simulink model "notch_filter"  (R2017a)
settings: Solver=VariableStepAuto  StartTime=0.0  StopTime=10  RelTol=1e-3
InitFcn:
  | r = 4700
  | c = 0.1e-6
  | fl = 1/(2*pi*r*c)
  | wl = 2*pi*fl
  | 
  | fn = 1526
  | wn = 2*pi*fn
  | 
  | t = 1.5e-4
libraries: dspstat3 x1, dspfdesign x1
settings Model: Creator=frede  LastModifiedBy=frede

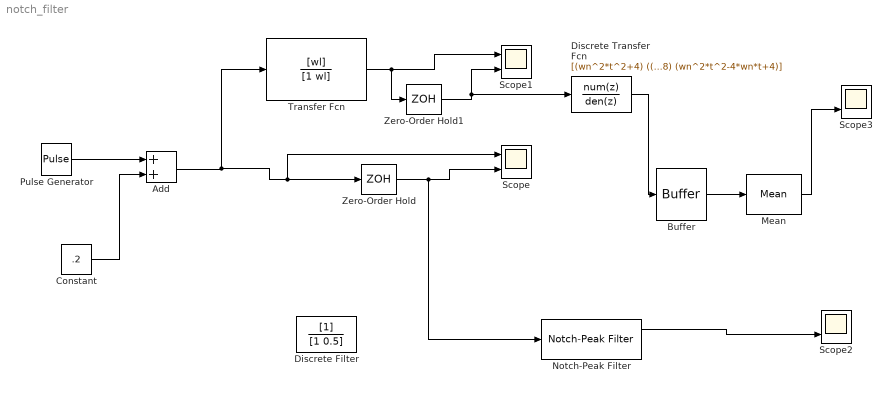
== system notch_filter ==
  Add : Sum
  Buffer : Buffer  N=230  OutputFrames=off
  Constant : Constant  Value=.2
  Discrete Transfer Fcn : DiscreteTransferFcn  Numerator=[(wn^2*t^2+4) ((wn^2*t-4)*2) (wn^2+4)]  Denominator=[(wn^2*t^2+4*wn*t+4) (2*wn^2*t^2-8) (wn^2*t^2-4*wn*t+4)]  SampleTime=t
  Discrete Filter : DiscreteFilter
  Mean : dspstat3/Mean  run=off  reset_popup=None  InputProcessing=Columns as channels (frame based)  directionMode=Each column  dimension=1  roiEnable=off  roiType=Rectangles  roiPortion=Entire ROI  roiOutput=Individual statistics for each ROI  roiFlag=off  outputDataTypeStr=Inherit: Same as accumulator  outputLastDataTypeStr=Inherit: Same as accumulator  outputMin=[]  outputMax=[]  roundingMode=Floor  overflowMode=off
  Notch-Peak Filter : dspfdesign/Notch-Peak Filter  Specification=Bandwidth and center frequency  Bandwidth=1000  QualityFactor=5  CenterFrequency=1526  BandwidthCoefficient=0.72654  CenterFrequencyCoefficient=0  Output=Notch and Peak  InheritSampleRate=off  SampleRate=44100  SimulateUsing=Code generation
      settings: SourceProductName=DSP System Toolbox  SourceProductBaseCode=DS
  Pulse Generator : DiscretePulseGenerator  PulseType=Time based  Period=1/1526  PulseWidth=50
  Scope{,1..3} (4 alike) : Scope  NumInputPorts=2
  Transfer Fcn : TransferFcn  Numerator=[wl]  Denominator=[1 wl]
  Zero-Order Hold : ZeroOrderHold  SampleTime=t
  Zero-Order Hold1 : ZeroOrderHold  SampleTime=t
  wires:
  Zero-Order Hold/1 -> Notch-Peak Filter/1, Scope/2
  Transfer Fcn/1 -> Zero-Order Hold1/1, Scope1/1
  Pulse Generator/1 -> Add/1
  Constant/1 -> Add/2
  Add/1 -> Scope/1, Zero-Order Hold/1, Transfer Fcn/1
  Zero-Order Hold1/1 -> Discrete Transfer Fcn/1, Scope1/2
  Notch-Peak Filter/1 -> Scope2/2
  Buffer/1 -> Mean/1
  Discrete Transfer Fcn/1 -> Buffer/1
  Mean/1 -> Scope3/2
